simulink model "adaptiv2"  (Simulink 7.8)
settings: Solver=ode45  StartTime=0.0  StopTime=2.5  RelTol=1e-3
values from neighbouring files (symbols this model uses):
  h = firpm(64,f,m)    [CFIR_1.m]    (also in adapt_filter1.m = adaptfilt.lms(ni,mu); adapt_filter2.m = adaptfilt.blms(ni,mu,1,36); adaptiv_2.m = [1 2 3 4 5 6 7 8 9 10]; adaptiv_3.m = [1 2 3 4 5 6 7 8 9 10])
  L = 24    [G722_1.m]    (also in adaptiv_2.m = length(h); adaptiv_3.m = length(h); audio_test1.m = 64; audio_test2.m = 64)
  m_noise = sqrt(noise)    [adaptiv_2.m]    (also in adaptiv_3.m; adaptiv_4.m; adaptiv_5.m; adaptiv_6.m)
  mu = 0.01    [adapt_filter1.m]    (also in adapt_filter2.m; adaptiv_2.m; adaptiv_3.m; adaptiv_4.m)
  Ts = 1/fs    (= 6.25e-05)    [G722_1.m]    (also in adaptiv_2.m = 0.001; adaptiv_3.m = 0.001; adaptiv_4.m = 0.001; adaptiv_5.m = 0.001)
libraries: dspobslib x1
settings Model: Creator=svenhoffmann  LastModifiedBy=josef  ExtModeAutoUpdateStatusClock=off
settings DataIOCC: SignalLoggingName=sigsOut
settings DebuggingCC: SaveWithParameterizedLinksMsg=none  SignalResolutionControl=TryResolveAllWithWarning  SolverPrmCheckMsg=none  MultiTaskDSMMsg=warning  MultiTaskCondExecSysMsg=none  StrictBusMsg=None
settings HardwareCC: TargetUnknown=on
settings RTWCC: IncludeERTFirstTime=on

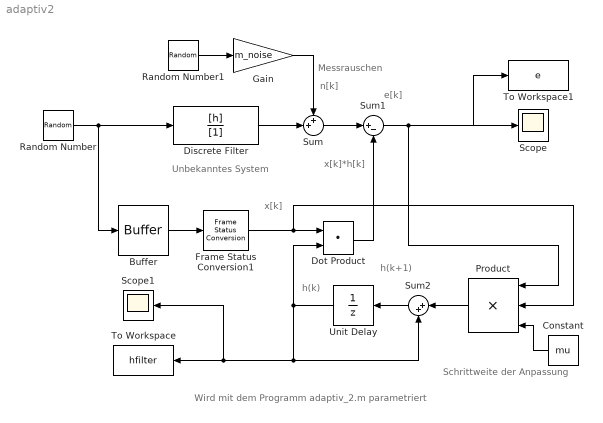
== system adaptiv2 ==
  note: Unbekanntes System
  note: Messrauschen
  note: e[k]
  note: x[k]
  note: Schrittweite der
      | Anpassung
  note: h(k+1)
  note: h(k)
  note: Wird mit dem Programm adaptiv_2.m parametriert
  note: n[k]
  note: x[k]*h[k]
  Buffer : Buffer  N=L  V=L-1
  Constant : Constant  Value=mu
  Discrete Filter : DiscreteFilter  Numerator=[h]  Denominator=[1]  SampleTime=Ts
  Dot Product : DotProduct  InputSameDT=on  OutDataTypeStr=Inherit: Inherit via internal rule
  Frame Status Conversion1 : dspobslib/Frame Status Conversion  growRefPort=off  outframe=Sample-based
  Gain : Gain  Gain=m_noise  SaturateOnIntegerOverflow=on  OutDataTypeStr=Inherit: Same as input  ParamDataTypeStr=Inherit: Same as input
  Product : Product  Inputs=3  SaturateOnIntegerOverflow=on  OutDataTypeStr=Inherit: Same as first input
  Random Number : RandomNumber  SampleTime=Ts
  Random Number1 : RandomNumber  Seed=13579  SampleTime=Ts
  Scope : Scope
      settings: YMin=-70000  YMax=100000
  Scope1 : Scope
      settings: YMin=-70000  YMax=100000
  Sum : Sum  Inputs=++|  SaturateOnIntegerOverflow=on
  Sum1 : Sum  Inputs=|+-  SaturateOnIntegerOverflow=on
  Sum2 : Sum  Inputs=|++  SaturateOnIntegerOverflow=on
  To Workspace : ToWorkspace  VariableName=hfilter  SampleTime=Ts  SaveFormat=Array
  To Workspace1 : ToWorkspace  VariableName=e  SampleTime=Ts  SaveFormat=Array
  Unit Delay : UnitDelay  X0=zeros(10,1)  SampleTime=Ts
  wires:
  Random Number/1 -> Discrete Filter/1, Buffer/1
  Buffer/1 -> Frame Status Conversion1/1
  Dot Product/1 -> Sum1/2
  Discrete Filter/1 -> Sum/2
  Random Number1/1 -> Gain/1
  Gain/1 -> Sum/1
  Sum/1 -> Sum1/1
  Sum2/1 -> Unit Delay/1
  Product/1 -> Sum2/1
  Sum1/1 -> Scope/1, Product/1, To Workspace1/1
  Constant/1 -> Product/3
  Frame Status Conversion1/1 -> Dot Product/1, Product/2
  Unit Delay/1 -> Dot Product/2, Sum2/2, To Workspace/1, Scope1/1
